simulink model "FinalECA"  (R2018a)
settings: Solver=FixedStepDiscrete  StartTime=0.0  StopTime=10.0  RelTol=1e-3
libraries: fuzblock x1
settings Model: Creator=Lakshya Tyagi  LastModifiedBy=laksh
settings OptimizationCC: DefaultParameterBehavior=Inlined  UseDivisionForNetSlopeComputation=on  UseFloatMulNetSlope=on  InlineInvariantSignals=on  PassReuseOutputArgsAs=Individual arguments  ZeroExternalMemoryAtStartup=off  ZeroInternalMemoryAtStartup=off  NoFixptDivByZeroProtection=on  EfficientFloat2IntCast=on  LifeSpan=1  OptimizeBlockOrder=speed  DifferentSizesBufferReuse=on
settings DebuggingCC: ParameterTunabilityLossMsg=error
settings HardwareCC: ProdLongLongMode=on
settings SFSimCC: MATLABDynamicMemAlloc=off
settings RTWCC: SystemTargetFile=ert.tlc  TemplateMakefile=ert_default_tmf  GenerateReport=on  IncludeHyperlinkInReport=on  LaunchReport=on  TargetLang=C++  GenerateTraceInfo=on  GenerateTraceReport=on  GenerateTraceReportSl=on  GenerateTraceReportSf=on  GenerateTraceReportEml=on
settings CodeAppCC: ForceParamTrailComments=on  IgnoreCustomStorageClasses=off  OperatorAnnotations=on  SimulinkDataObjDesc=on  SFDataObjDesc=on  CustomSymbolStrGlobalVar=rt$N$M  CustomSymbolStrType=$N$M  CustomSymbolStrFcn=$N$M$F  CustomSymbolStrMacro=$N$M  InsertBlockDesc=on
settings ERTTargetCC: TargetLangStandard=C++03 (ISO)  GenerateSampleERTMain=on  IncludeMdlTerminateFcn=off  CombineSignalStateStructs=on  SupportAbsoluteTime=off  MultiInstanceERTCode=on  CodeInterfacePackaging=C++ class  SupportComplex=off  SupportNonInlinedSFcns=on  InlinedParameterPlacement=NonHierarchical  RootIOFormat=Structure reference  ERTCustomFileTemplate=example_file_process.tlc  ERTFilePackagingFormat=CompactWithDataFile

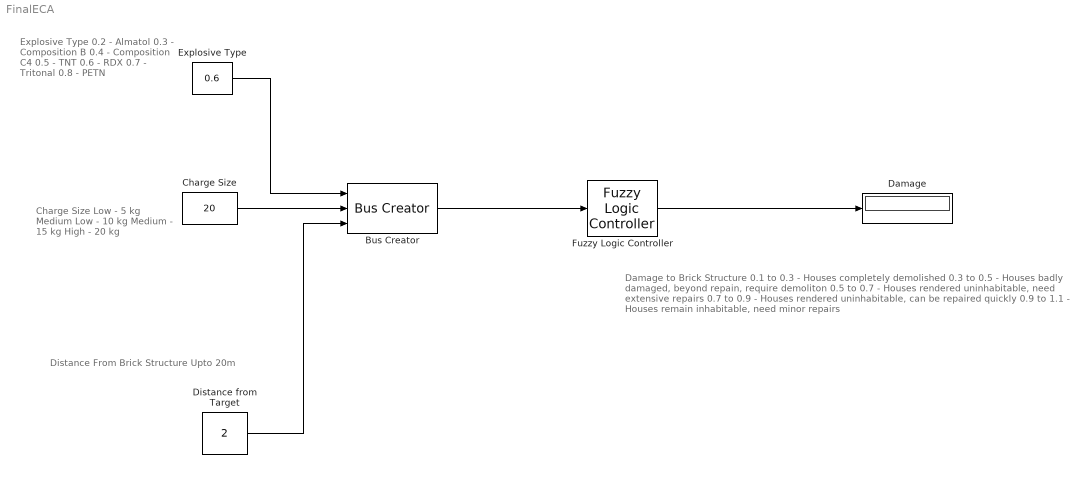
== system FinalECA ==
  note: Damage to Brick Structure
      |
      | 0.1 to 0.3 - Houses completely demolished
      | 0.3 to 0.5 - Houses badly damaged, beyond repain, require demoliton
      | 0.5 to 0.7 - Houses rendered uninhabitable, need extensive repairs
      | 0.7 to 0.9 - Houses rendered uninhabitable, can be repaired quickly
      | 0.9 to 1.1 - Houses remain inhabitable, need minor repairs
  note: Distance From Brick Structure
      |
      | Upto 20m
  note: Charge Size
      |
      | Low - 5 kg
      | Medium Low - 10 kg
      | Medium - 15 kg
      | High - 20 kg
  note: Explosive Type
      | 0.2 - Almatol
      | 0.3 - Composition B
      | 0.4 - Composition C4
      | 0.5 - TNT
      | 0.6 - RDX
      | 0.7 - Tritonal
      | 0.8 - PETN
  Bus Creator : BusCreator  Inputs=3
  Charge Size : Constant  Value=20
  Damage : Display
  Distance from Target : Constant  Value=2
  Explosive Type : Constant  Value=0.6
  Fuzzy Logic Controller : fuzblock/Fuzzy Logic  Controller  FIS='ECA.fis'  OutputSampleNumber=101  DataType=double  FuzzifiedInputs=off  RuleFiringStrengths=off  RuleOutputs=off  AggregatedOutputs=off  SimulateUsing=Interpreted execution  OutOfRangeInputValueMessage=warning  NoRuleFiredMessage=warning  EmptyOutputFuzzySetMessage=warning
  wires:
  Explosive Type/1 -> Bus Creator/1
  Charge Size/1 -> Bus Creator/2
  Distance from Target/1 -> Bus Creator/3
  Bus Creator/1 -> Fuzzy Logic Controller/1
  Fuzzy Logic Controller/1 -> Damage/1
